simulink subsystem "Fit_Poly_2_Waypoints"  (R2022b)
settings: Solver=VariableStepAuto  StartTime=0.0  StopTime=10.0  RelTol=1e-3
settings Model: Creator=User  LastModifiedBy=User

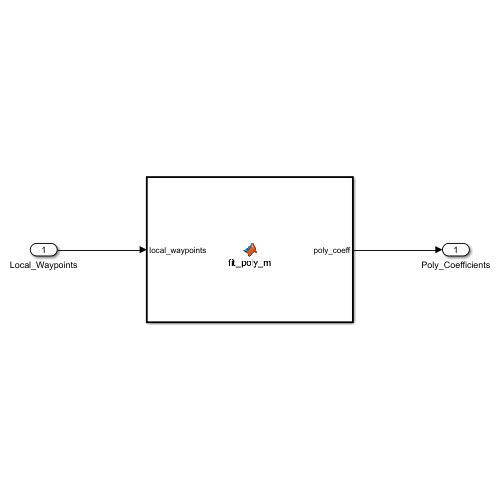
[thumbnail: Simulink's stored preview of the top-level diagram]
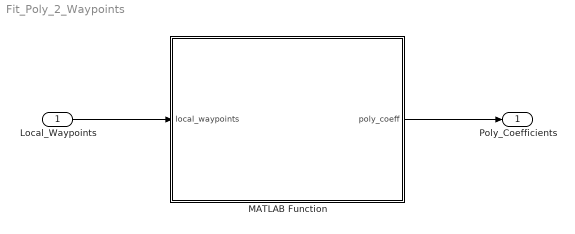
== system Fit_Poly_2_Waypoints ==
  Local_Waypoints : Inport
  MATLAB Function : MATLAB Function  TreatAsAtomicUnit=on
  Poly_Coefficients : Outport
  wires:
  Local_Waypoints/1 -> MATLAB Function/1(local_waypoints)
  MATLAB Function/1(poly_coeff) -> Poly_Coefficients/1

== matlab function Fit_Poly_2_Waypoints/MATLAB Function ==
  data: local_waypoints input; poly_coeff output
function poly_coeff = fit_poly_m(local_waypoints)
     poly_coeff = fit_poly(local_waypoints);
    
end
